simulink model "EMB_CVT"  (R2023a)
settings: Solver=VariableStepAuto  StartTime=0.0  StopTime=200.0  RelTol=1e-3
undefined symbols (not defined in the file): controller, sigbuilder_block
libraries: fl_lib x19, sdl_lib x9, nesl_utility x8, simulink x1, slpidlib x1, autolibshared x1, batteryecm_lib x1, BatteryEstimators x1, ee_lib x1
settings Model: Creator=Rohan  LastModifiedBy=Rohan

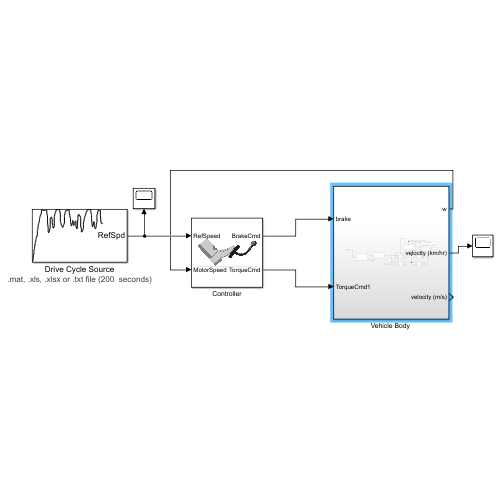
[thumbnail: Simulink's stored preview of the top-level diagram]
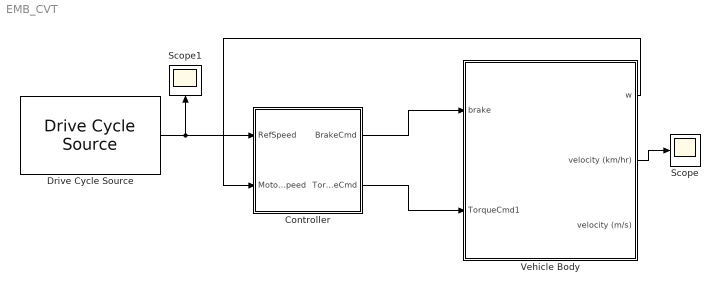
== system EMB_CVT ==
  Controller : Subsystem  VariantControl=a==1
      mask Display: image('$imagefile'); % Use "Edit Image" on toolstrip to change.
  Drive Cycle Source : autolibshared/Drive Cycle Source  cycleVar=.mat, .xls, .xlsx or .txt file  fileVar=D:\BAJA Battery\Day2 (1)\Day2\1_drive_cycle\driveCycleb.mat  tfinal="200  seconds"  cycleRepeat=off  outAccPort=off  outGearPort=off  gearList=No gear data  t_wot1=5  xdot_woto=0  xdot_wot1=30  t_wot2=20  xdot_wot2=0  t_wotend=30  srcUnit=m/s  outUnit=m/s  srcAccUnit=m/s/s  outAccUnit=m/s^2  dt=0  aMode=1  faultOption=off  velBnd=2  velBndUnit=mph  inUnit=m/s  timeBnd=1  failOption=off  stopSim=off  maxFaultCnt=10  maxFaultTime=2  maxTotFaultTime=15  traceOption=off  dtTrace=1  traceWindow=10  lastDCname=Custom Data Set  lastOutUnit=mph  lastDT=0  lastTB=1  lastSB=2  forceCalcBound=off
  Scope : Scope
  Scope1 : Scope
  "Vehicle Body " : Subsystem
  wires:
  Controller/2(TorqueCmd) -> "Vehicle Body "/2(TorqueCmd1)
  "Vehicle Body "/2(velocity (km/hr)) -> Scope/1
  Controller/1(BrakeCmd) -> "Vehicle Body "/1(brake)
  Drive Cycle Source/1 -> Controller/1(RefSpeed), Scope1/1
  "Vehicle Body "/1(w) -> Controller/2(MotorSpeed)

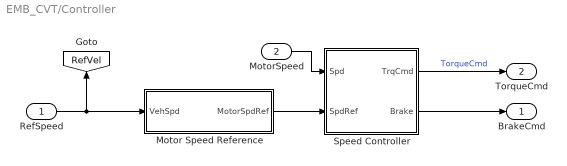
== system EMB_CVT/Controller ==
  RefSpeed : Inport
  MotorSpeed : Inport  Port=2
  Motor Speed Reference : Subsystem
  Speed Controller : Subsystem
      settings: PortSchema="{\"entries\":[{\"content\":{\"sides\":[{\"content\":{\"connectorIds\":[\"Out1\",\"Out2\"]},\"type\":\"ConnectorPlacement.EquallySpacedRectSide\",\"uuid\":\"12b9f2c9-2b28-451b-ad36-7fe4150db485\"},{\"content\":{\"connectorIds\":[\"In1\",\"In2\"],\"side\":\"RIGHT\"},\"type\":\"ConnectorPlacement.EquallySpacedRectSide\",\"uuid\":\"c0fdf9a4-483a-4ddc-b663-6299fcc79327\"},{\"content\":{\"connectorIds\":[],\"side\":\"TOP\"},\"type\":\"ConnectorPlacement.EquallySpacedRectSide\",\"uuid\":\"3f20082e-8487-45e3-9fd7-d6d75741df4d\"}]},\"type\":\"ConnectorPlacement.EquallySpacedConnector\",\"uuid\":\"9361cdd3-74d8-46ee-ae7f-e2dde5d31ed1\"}],\"packageUris\":[\"http://schema.mathworks.com/mf0/Connector/R2020b\"],\"version\":\"1.0\"}"
  BrakeCmd : Outport
  TorqueCmd : Outport  Port=2
  tag scope: RefVel=global
  wires:
  Speed Controller/2(Brake) -> BrakeCmd/1
  Motor Speed Reference/1(MotorSpdRef) -> Speed Controller/2(SpdRef)
  MotorSpeed/1 -> Speed Controller/1(Spd)
  Speed Controller/1(TrqCmd) -> TorqueCmd/1  "TorqueCmd"
  RefSpeed/1 -> Motor Speed Reference/1(VehSpd), [RefVel]

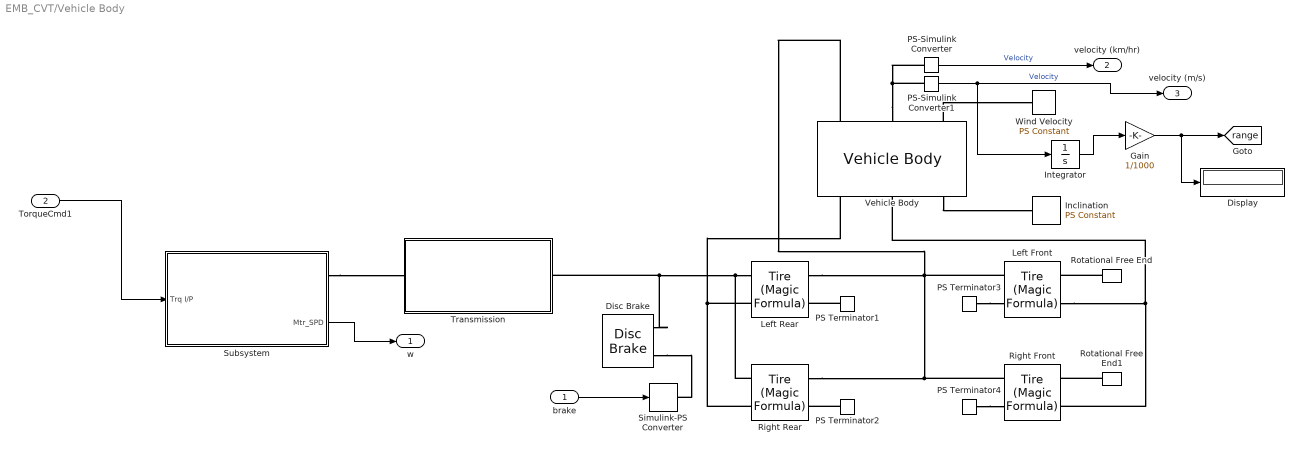
== system EMB_CVT/Vehicle Body  ==
  brake : Inport
  TorqueCmd1 : Inport  Port=2
  Disc Brake : sdl_lib/Brakes & Detents/Rotational/Disc Brake  r_mean=brake.padRadius mm  bore=brake.cylinderBore mm  n_pads=2  thermal_port=simscape.enum.thermaleffects.omit  mu_static=brake.sf  mu_coulomb=brake.cf  temperature_TLU=[280, 300, 320] K  mu_static_TLU=[.9, .8, .7]  mu_coulomb_TLU=[.8, .7, .6]  brkwy_vel=brake.frictionVel rad/s  visc_coef=0 N*m*s/rad  enable_faults=simscape.enum.onoff.off  faulted_pressure=0 bar  external_fault=simscape.enum.onoff.off  temporal_fault=simscape.enum.onoff.off  fault_time=5 s  report_fault=simscape.enum.assert.action.none  thermal_mass=50 kJ/K  temperature_specify=off  temperature_priority=High  temperature=300 K  temperature_nominal_specify=off  temperature_nominal_unit=K  temperature_nominal_value=1
  Display : Display
  Gain : Gain  Gain=1/1000
  Inclination : fl_lib/Physical Signals/Sources/PS Constant  constant=0
  Integrator : Integrator
  Left Front : sdl_lib/Tires & Vehicles/Tire (Magic Formula)  parameterization=sdl.enum.magic_tire_model.constant  F_z1=3000 N  F_x1=3500 N  kappa1=10  B_m=vehicle.tireBCoeff  C_m=vehicle.tireCCoeff  D_m=vehicle.tireDCoeff  E_m=vehicle.tireECoeff  fz0=4000 N  p_Cx=1.685  p_Dx=[1.21, -.037]  p_Ex=[.344, .095, -.02, 0]  p_Kx=[21.51, -.163, .245]  p_Hx=[-.002, .002]  p_Vx=[0, 0]  rolling_radius_model=sdl.enum.RollingRadiusParameterization.Constant  r_e=vehicle.tireRollingRadius m  r_0=0.3 m  breff=8.39  dreff=0.26  freff=0.074  q_re0=0.99  q_v1=0.008  longvl=17 m/s  cz=5e5 N/m  model_resistance=1  resistance_model=1  coeff=0.005  p_tire=250e3 Pa  alpha=-0.003  beta=0.97  coeff_a=84e-4  coeff_b=6.2e-4 s/m  coeff_c=1.6e-4 s^2/m^2  p_tire0=240e3 Pa  fz0_resistance=4000 N  vH0=16 m/s  q_Sy=[.0082, 0, .0014, .001, 0, 0, 1.08, -.5]  v_thr=0.001 m/s  enable_scaling_coefficients=false  lfzO=1  lcx=1  lmux=1  lex=1  lkx=1  lhx=1  lvx=1  lmy=1  model_compliance=0  stiffness=1e6 N/m  damping=1000 N/(m/s)  model_inertia=1  inertia=1e-2 kg*m^2  initial_velocity=0 rpm  vxlow=0.1 m/s  v_tr_thr=0.1*(0.1) m/s  kpumin=-1e5  kpumax=1e5
  Left Rear : sdl_lib/Tires & Vehicles/Tire (Magic Formula)  parameterization=sdl.enum.magic_tire_model.constant  F_z1=3000 N  F_x1=3500 N  kappa1=10  B_m=vehicle.tireBCoeff  C_m=vehicle.tireCCoeff  D_m=vehicle.tireDCoeff  E_m=vehicle.tireECoeff  fz0=4000 N  p_Cx=1.685  p_Dx=[1.21, -.037]  p_Ex=[.344, .095, -.02, 0]  p_Kx=[21.51, -.163, .245]  p_Hx=[-.002, .002]  p_Vx=[0, 0]  rolling_radius_model=sdl.enum.RollingRadiusParameterization.Constant  r_e=vehicle.tireRollingRadius m  r_0=0.3 m  breff=8.39  dreff=0.26  freff=0.074  q_re0=0.99  q_v1=0.008  longvl=17 m/s  cz=5e5 N/m  model_resistance=1  resistance_model=1  coeff=0.005  p_tire=250e3 Pa  alpha=-0.003  beta=0.97  coeff_a=84e-4  coeff_b=6.2e-4 s/m  coeff_c=1.6e-4 s^2/m^2  p_tire0=240e3 Pa  fz0_resistance=4000 N  vH0=16 m/s  q_Sy=[.0082, 0, .0014, .001, 0, 0, 1.08, -.5]  v_thr=0.001 m/s  enable_scaling_coefficients=false  lfzO=1  lcx=1  lmux=1  lex=1  lkx=1  lhx=1  lvx=1  lmy=1  model_compliance=0  stiffness=1e6 N/m  damping=1000 N/(m/s)  model_inertia=1  inertia=1e-2 kg*m^2  initial_velocity=0 rpm  vxlow=0.1 m/s  v_tr_thr=0.1*(0.1) m/s  kpumin=-1e5  kpumax=1e5
  PS Terminator{1..4} (4 alike) : fl_lib/Physical Signals/Sinks/PS Terminator
  PS-Simulink Converter : nesl_utility/PS-Simulink Converter  PhysicalDomain=network_engine_domain  SubClassName=ps_output  LeftPortType=input  RightPortType=output  PseudoPeriodic=off  Frequencies=[]  VectorFormat=1-D array  Unit=km/hr  AffineConversion=off
  PS-Simulink Converter1 : nesl_utility/PS-Simulink Converter  PhysicalDomain=network_engine_domain  SubClassName=ps_output  LeftPortType=input  RightPortType=output  PseudoPeriodic=off  Frequencies=[]  VectorFormat=1-D array  Unit=m/s  AffineConversion=off
  Right Front : sdl_lib/Tires & Vehicles/Tire (Magic Formula)  parameterization=sdl.enum.magic_tire_model.constant  F_z1=3000 N  F_x1=3500 N  kappa1=10  B_m=vehicle.tireBCoeff  C_m=vehicle.tireCCoeff  D_m=vehicle.tireDCoeff  E_m=vehicle.tireECoeff  fz0=4000 N  p_Cx=1.685  p_Dx=[1.21, -.037]  p_Ex=[.344, .095, -.02, 0]  p_Kx=[21.51, -.163, .245]  p_Hx=[-.002, .002]  p_Vx=[0, 0]  rolling_radius_model=sdl.enum.RollingRadiusParameterization.Constant  r_e=vehicle.tireRollingRadius m  r_0=0.3 m  breff=8.39  dreff=0.26  freff=0.074  q_re0=0.99  q_v1=0.008  longvl=17 m/s  cz=5e5 N/m  model_resistance=1  resistance_model=1  coeff=0.005  p_tire=250e3 Pa  alpha=-0.003  beta=0.97  coeff_a=84e-4  coeff_b=6.2e-4 s/m  coeff_c=1.6e-4 s^2/m^2  p_tire0=240e3 Pa  fz0_resistance=4000 N  vH0=16 m/s  q_Sy=[.0082, 0, .0014, .001, 0, 0, 1.08, -.5]  v_thr=0.001 m/s  enable_scaling_coefficients=false  lfzO=1  lcx=1  lmux=1  lex=1  lkx=1  lhx=1  lvx=1  lmy=1  model_compliance=0  stiffness=1e6 N/m  damping=1000 N/(m/s)  model_inertia=1  inertia=1e-2 kg*m^2  initial_velocity=0 rpm  vxlow=0.1 m/s  v_tr_thr=0.1*(0.1) m/s  kpumin=-1e5  kpumax=1e5
  Right Rear : sdl_lib/Tires & Vehicles/Tire (Magic Formula)  parameterization=sdl.enum.magic_tire_model.constant  F_z1=3000 N  F_x1=3500 N  kappa1=10  B_m=vehicle.tireBCoeff  C_m=vehicle.tireCCoeff  D_m=vehicle.tireDCoeff  E_m=vehicle.tireECoeff  fz0=4000 N  p_Cx=1.685  p_Dx=[1.21, -.037]  p_Ex=[.344, .095, -.02, 0]  p_Kx=[21.51, -.163, .245]  p_Hx=[-.002, .002]  p_Vx=[0, 0]  rolling_radius_model=sdl.enum.RollingRadiusParameterization.Constant  r_e=vehicle.tireRollingRadius m  r_0=0.3 m  breff=8.39  dreff=0.26  freff=0.074  q_re0=0.99  q_v1=0.008  longvl=17 m/s  cz=5e5 N/m  model_resistance=1  resistance_model=1  coeff=0.005  p_tire=250e3 Pa  alpha=-0.003  beta=0.97  coeff_a=84e-4  coeff_b=6.2e-4 s/m  coeff_c=1.6e-4 s^2/m^2  p_tire0=240e3 Pa  fz0_resistance=4000 N  vH0=16 m/s  q_Sy=[.0082, 0, .0014, .001, 0, 0, 1.08, -.5]  v_thr=0.001 m/s  enable_scaling_coefficients=false  lfzO=1  lcx=1  lmux=1  lex=1  lkx=1  lhx=1  lvx=1  lmy=1  model_compliance=0  stiffness=1e6 N/m  damping=1000 N/(m/s)  model_inertia=1  inertia=1e-2 kg*m^2  initial_velocity=0 rpm  vxlow=0.1 m/s  v_tr_thr=0.1*(0.1) m/s  kpumin=-1e5  kpumax=1e5
  Rotational Free End : fl_lib/Mechanical/Rotational Elements/Rotational Free End  w_specify=off  w_priority=None  w=0 rad/s  w_nominal_specify=off  w_nominal_unit=rad/s  w_nominal_value=1
  Rotational Free End1 : fl_lib/Mechanical/Rotational Elements/Rotational Free End  w_specify=off  w_priority=None  w=0 rad/s  w_nominal_specify=off  w_nominal_unit=rad/s  w_nominal_value=1
  Simulink-PS Converter : nesl_utility/Simulink-PS Converter  PhysicalDomain=network_engine_domain  SubClassName=ps_input  LeftPortType=input  RightPortType=output  PseudoPeriodic=off  Frequencies=[]  NoiseDistribution=none  NoiseParameters=[]  Unit=N/m^2  AffineConversion=off  FilteringAndDerivatives=filter  SimscapeFilterOrder=2  InputFilterTimeConstant=0.001  UdotUserProvided=1
  Subsystem : Subsystem
      settings: PortSchema="{\"entries\":[{\"content\":{\"sides\":[{\"content\":{\"connectorIds\":[\"In1\"]},\"type\":\"ConnectorPlacement.EquallySpacedRectSide\",\"uuid\":\"a8b1f416-e8b0-4c0a-8f46-8c70d4c0ad6f\"},{\"content\":{\"connectorIds\":[\"RConn1\",\"Out1\"],\"side\":\"RIGHT\"},\"type\":\"ConnectorPlacement.EquallySpacedRectSide\",\"uuid\":\"f31562b3-4fb8-47fa-b272-1277153c0f5f\"},{\"content\":{\"side\":\"TOP\"},\"type\":\"ConnectorPlacement.EquallySpacedRectSide\",\"uuid\":\"367d0b97-d35b-412e-9cb2-5cff6624febc\"}]},\"type\":\"ConnectorPlacement.EquallySpacedConnector\",\"uuid\":\"bebd6450-d495-493e-a389-2977d92ebb5e\"}],\"packageUris\":[\"http://schema.mathworks.com/mf0/Connector/R2020b\"],\"version\":\"1.0\"}"
  Transmission : Subsystem
  Vehicle Body : sdl_lib/Tires & Vehicles/Vehicle Body  mass=vehicle.mass kg  n_w=vehicle.numAxle  x_f=vehicle.cgFrontAxle m  x_r=vehicle.cgRearAxle m  y_c=vehicle.cgGround m  mass_var=simscape.enum.onoff.off  g=9.81 m/s^2  liftoff_warning=0  area=.735482 m^2  Cd=1.92  rho=1.18 kg/m^3  model_pitch=0  inertia=4000 kg*m^2  suspension_model=1  k_f=1e4 N/m  b_f=1e4 N/(m/s)  k_r=1e4 N/m  b_r=1e4 N/(m/s)  k_f_TLU=[-2000, -1000, 0, 1000, 2000] N  x_f_TLU=[-.4, -.2, 0, .2, .4] m  b_f_TLU=[-200, -100, 0, 100, 200] N  v_f_TLU=[-4, -2, 0, 2, 4] m/s  k_r_TLU=[-2000, -1000, 0, 1000, 2000] N  x_r_TLU=[-.4, -.2, 0, .2, .4] m  b_r_TLU=[-200, -100, 0, 100, 200] N  v_r_TLU=[-4, -2, 0, 2, 4] m/s  interp_method=simscape.enum.interpolation.linear  extrap_method=simscape.enum.extrapolation.linear  model_hardstop=0  upper_bound_f=.25 m  lower_bound_f=-.25 m  stop_k_f=1e6 N/m  stop_b_f=150 N/(m/s)  upper_bound_r=.25 m  lower_bound_r=-.25 m  stop_k_r=1e6 N/m  stop_b_r=150 N/(m/s)  initial_pitch=0 rad  initial_pitch_rate=0 rad/s  v_specify=on  v_priority=High  v=0 m/s  v_nominal_specify=off  v_nominal_unit=m/s  v_nominal_value=1
  Wind Velocity : fl_lib/Physical Signals/Sources/PS Constant  constant=0
  w : Outport
  velocity (km/hr) : Outport  Port=2
  velocity (m/s) : Outport  Port=3
  tag scope: range=global
  wires:
  Integrator/1 -> Gain/1
  PS-Simulink Converter1/1 -> Integrator/1, velocity (m/s)/1  "Velocity"
  brake/1 -> Simulink-PS Converter/1
  PS-Simulink Converter/1 -> velocity (km/hr)/1  "Velocity"
  Gain/1 -> Display/1, [range]
  TorqueCmd1/1 -> Subsystem/1(Trq I/P)
  Subsystem/1(Mtr_SPD) -> w/1
  connections:
  Vehicle Body/RConn2 -- Right Front/LConn1 -- Left Front/LConn1
  Vehicle Body/LConn2 -- PS-Simulink Converter/LConn1 -- PS-Simulink Converter1/LConn1
  Right Front/RConn2 -- Vehicle Body/LConn1 -- Left Rear/RConn2 -- Left Front/RConn2 -- Right Rear/RConn2
  Vehicle Body/RConn1 -- Left Rear/LConn1 -- Right Rear/LConn1
  PS Terminator1/LConn1 -- Left Rear/RConn1
  Vehicle Body/LConn3 -- Wind Velocity/RConn1
  Vehicle Body/RConn3 -- Inclination/RConn1
  Disc Brake/LConn1 -- Simulink-PS Converter/RConn1
  PS Terminator3/LConn1 -- Left Front/RConn1
  PS Terminator2/LConn1 -- Right Rear/RConn1
  Rotational Free End/LConn1 -- Left Front/LConn2
  PS Terminator4/LConn1 -- Right Front/RConn1
  Rotational Free End1/LConn1 -- Right Front/LConn2
  Right Rear/LConn2 -- Disc Brake/LConn2 -- Transmission/RConn1 -- Left Rear/LConn2
  Subsystem/RConn1 -- Transmission/LConn1

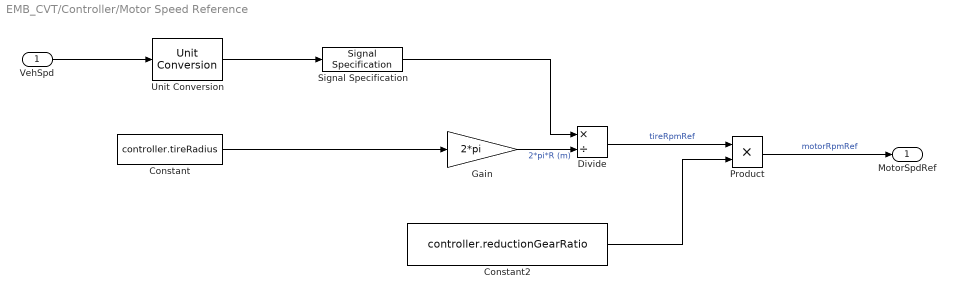
== system EMB_CVT/Controller/Motor Speed Reference ==
  VehSpd : Inport  Unit=km/hr
  Constant : Constant  Value=controller.tireRadius
  Constant2 : Constant  Value=controller.reductionGearRatio
  Divide : Product  Inputs=*/
  Gain : Gain  Gain=2*pi
  Product : Product
  Signal Specification : SignalSpecification  Unit=m/min
  Unit Conversion : UnitConversion
  MotorSpdRef : Outport  Unit=rpm  VectorParamsAs1DForOutWhenUnconnected=off
  wires:
  Product/1 -> MotorSpdRef/1  "motorRpmRef"
  Constant2/1 -> Product/2
  Divide/1 -> Product/1  "tireRpmRef"
  Gain/1 -> Divide/2  "2*pi*R (m)"
  Signal Specification/1 -> Divide/1
  Unit Conversion/1 -> Signal Specification/1
  VehSpd/1 -> Unit Conversion/1
  Constant/1 -> Gain/1

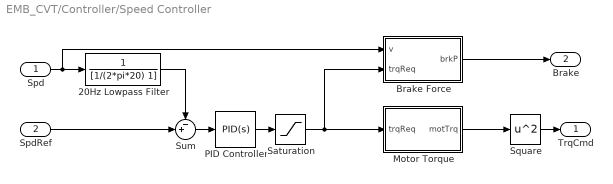
== system EMB_CVT/Controller/Speed Controller ==
  Spd : Inport  Unit=rpm
  SpdRef : Inport  Port=2  Unit=rpm
  20Hz Lowpass Filter : TransferFcn  Denominator=[1/(2*pi*20) 1]
  Brake Force : Subsystem
  Motor Torque : Subsystem
  PID Controller : slpidlib/PID Controller  Controller=PID  Form=Parallel  TimeDomain=Continuous-time  UseExternalTs=off  SampleTime=-1  IntegratorMethod=Forward Euler  FilterMethod=Forward Euler  ControllerParametersSource=internal  P=1  I=1  UseKiTs=off  D=0  N=100  UseFilter=on  TunerSelectOption=Transfer Function Based (PID Tuner App)  InitialConditionSource=internal  InitialConditionForIntegrator=0  InitialConditionForFilter=0  DifferentiatorICPrevScaledInput=0  ExternalReset=none  TrackingMode=off  Kt=1  LimitOutput=off  SatLimitsSource=internal  UpperSaturationLimit=inf  LowerSaturationLimit=-inf  LinearizeAsGain=on  AntiWindupMode=none  Kb=1  LimitIntegrator=off  UpperIntegratorSaturationLimit=inf  LowerIntegratorSaturationLimit=-inf  POutMin=[]  POutMax=[]  IOutMin=[]  IOutMax=[]  DOutMin=[]  DOutMax=[]  NOutMin=[]  NOutMax=[]  SumOutMin=[]  SumOutMax=[]  SaturationOutMin=[]  SaturationOutMax=[]  PParamMin=[]  PParamMax=[]  IParamMin=[]  IParamMax=[]  DParamMin=[]  DParamMax=[]  NParamMin=[]  NParamMax=[]  KbParamMin=[]  KbParamMax=[]  KtParamMin=[]  KtParamMax=[]  KbOutMin=[]  KbOutMax=[]  KtOutMin=[]  KtOutMax=[]  IntegratorOutMin=[]  IntegratorOutMax=[]  FilterOutMin=[]  FilterOutMax=[]  SumI1OutMin=[]  SumI1OutMax=[]  SumI2OutMin=[]  SumI2OutMax=[]  SumI3OutMin=[]  SumI3OutMax=[]  SumI4OutMin=[]  SumI4OutMax=[]  SumDOutMin=[]  SumDOutMax=[]  DifferentiatorOutMin=[]  DifferentiatorOutMax=[]  FilterDiffOutCoefMin=[]  FilterDiffOutCoefMax=[]  ReciprocalOutMin=[]  ReciprocalOutMax=[]  SumDenOutMin=[]  SumDenOutMax=[]  SumNumOutMin=[]  SumNumOutMax=[]  DivideOutMin=[]  DivideOutMax=[]  UdiffTsProdOutMin=[]  UdiffTsProdOutMax=[]  NTsProdOutMin=[]  NTsProdOutMax=[]  UintegralTsProdOutMin=[]  UintegralTsProdOutMax=[]  UngainTsProdOutMin=[]  UngainTsProdOutMax=[]  ClampingZeroOutDataTypeStr=Inherit: Inherit via back propagation  ClampingZeroOutMin=[]  ClampingZeroOutMax=[]  FilterDenConstantOutDataTypeStr=Inherit: Inherit via back propagation  FilterDenConstantOutMin=[]  FilterDenConstantOutMax=[]  PCopyOutDataTypeStr=Inherit: Inherit via back propagation  PCopyOutMin=[]  PCopyOutMax=[]  NCopyOutDataTypeStr=Inherit: Inherit via back propagation  NCopyOutMin=[]  NCopyOutMax=[]  IntegratorContinuousStateAttributes=''  IntegratorStateMustResolveToSignalObject=off  IntegratorRTWStateStorageClass=Auto  FilterContinuousStateAttributes=''  FilterStateMustResolveToSignalObject=off  FilterRTWStateStorageClass=Auto  ParallelPVariant=InternalParameters  IdealPVariant=Disabled  IVariant=InternalParameters  DVariant=InternalParameters  IntegratorVariant=Continuous  SatVariant=Disabled  AWVariant=Passthrough  PCopyVariant=Disabled  TRVariant=Disabled  FdbkBlocksVariant=Forward  IdealPFdbkVariant=Disabled  SatFdbkVariant=Disabled  DerivativeFilterVariant=ContFilter  NVariant=InternalParameters  NCopyVariant=Disabled  FilterICVariant=InternalICsFilter  IntegratorICVariant=InternalICs  ExternalResetVariant=Disabled  TRSumVariant=Passthrough  SumFdbkVariant=Disabled  SumVariant=Sum_PID  TsampFilterVariant=InternalTs  TsampNgainVariant=Passthrough  TsampIntegralVariant=Disabled_SignalSpec  ExternalSaturationOutDataTypeStr=Inherit: Same as second input
  Saturation : Saturate  UpperLimit=35  LowerLimit=-35
      settings: AttributesFormatString=|
      | %<UpperLimit>
      | %<LowerLimit>
  Square : Math  Operator=square
  Sum : Sum  Inputs=-+|
  TrqCmd : Outport  Unit=N*m  VectorParamsAs1DForOutWhenUnconnected=off
      settings: AttributesFormatString=%<Unit>
  Brake : Outport  Port=2  VectorParamsAs1DForOutWhenUnconnected=off
      settings: AttributesFormatString=%<Unit>
  wires:
  Saturation/1 -> Motor Torque/1(trqReq), Brake Force/2(trqReq)
  SpdRef/1 -> Sum/2
  PID Controller/1 -> Saturation/1
  Sum/1 -> PID Controller/1
  Spd/1 -> Brake Force/1(v), 20Hz Lowpass Filter/1
  Brake Force/1(brkP) -> Brake/1
  20Hz Lowpass Filter/1 -> Sum/1
  Square/1 -> TrqCmd/1
  Motor Torque/1(motTrq) -> Square/1

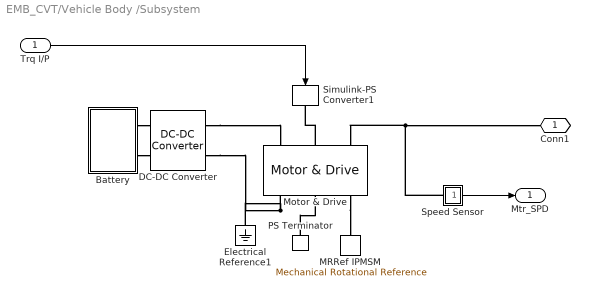
== system EMB_CVT/Vehicle Body /Subsystem ==
  Trq I/P : Inport
  Battery : Subsystem
  DC-DC Converter : ee_lib/Semiconductors & Converters/Converters/DC-DC Converter  Vref_option=ee.enum.converters.voltageref.internal  v_ref=converter.outputVoltage V  P_rated=converter.outputPower kW  droop_enabled=true  droop_param=ee.enum.converters.droop.percent  droop=0.1 V/A  droop_percent=converter.droopPercent  Vref_droop=10 V  reversible=ee.enum.converters.directionality.bidirectional  G_diode=1e-8 1/Ohm  P_fixed=1 W  losses_option=ee.enum.converters.lossesOption.proportionalToSquaredCurrent  eff_rated=80  tableOption=ee.enum.converters.lossTableOptionThermal.currentTemp  i_eff_vec=[-2, -1, 1, 2] A  v_eff_vec=[15, 30, 45] V  eff_vec=[66, 76, 80, 74]  eff_2D_table=[66, 66, 66; 76, 76, 76; 80, 80, 80; 74, 74, 74]  model_dynamics=ee.enum.converters.dynamics.no  tau=0.02 s  v_ini=10 V  v1_min=1 V  R1=1000 Ohm  R2=1000 Ohm  enable_fault=simscape.enum.onoff.off  fault_condition=ee.enum.faults.faultInputCondition.greaterThan  fault_threshold=0.5  T_eff_vec=[280, 300, 320] K  eff_3D_table=repmat([66; 76; 80; 74], 1, 3, 3)  thermal_mass=100 J/K  initial_temperature=298.15 K
      settings: InternalSimscapePortConfiguration="{\"Bottom\":[],\"Left\":[{\"id\":\"p1\",\"label\":\"1+\",\"type\":\"foundation.electrical.electrical\"},{\"id\":\"n1\",\"label\":\"1-\",\"type\":\"foundation.electrical.electrical\"}],\"Right\":[{\"id\":\"p2\",\"label\":\"2+\",\"type\":\"foundation.electrical.electrical\"},{\"id\":\"n2\",\"label\":\"2-\",\"type\":\"foundation.electrical.electrical\"}],\"Top\":[]}"
  Electrical Reference1 : fl_lib/Electrical/Electrical Elements/Electrical Reference
  MRRef IPMSM : fl_lib/Mechanical/Rotational Elements/Mechanical Rotational Reference
  Motor & Drive : sdl_lib/Engines & Motors/Motor & Drive  torque_max=motor.maxTorque N*m  power_max=motor.maxPower kW  Tc=motor.torqueTc s  eff=motor.overallEfficiency  w_eff=motor.speedatEff rpm  T_eff=motor.torqueatEff N*m  thermal_port=simscape.enum.thermaleffects.omit  thermal_mass=10 J/K  temperature_specify=on  temperature_priority=High  temperature=5 degC  temperature_nominal_specify=off  temperature_nominal_unit=K  temperature_nominal_value=1
      settings: InternalSimscapePortConfiguration="{\"Bottom\":[],\"Left\":[{\"id\":\"Vp\",\"label\":\"+\",\"type\":\"foundation.electrical.electrical\"},{\"id\":\"Tr\",\"label\":\"Tr\",\"type\":\"input\"},{\"id\":\"R\",\"label\":\"R\",\"type\":\"foundation.mechanical.rotational.rotational\"}],\"Right\":[{\"id\":\"Vm\",\"label\":\"-\",\"type\":\"foundation.electrical.electrical\"},{\"id\":\"Omega\",\"label\":\"w\",\"type\":\"output\"},{\"id\":\"C\",\"label\":\"C\",\"type\":\"foundation.mechanical.rotational.rotational\"}],\"Top\":[]}"
  PS Terminator : fl_lib/Physical Signals/Sinks/PS Terminator
  Simulink-PS Converter1 : nesl_utility/Simulink-PS Converter  PhysicalDomain=network_engine_domain  SubClassName=ps_input  LeftPortType=input  RightPortType=output  PseudoPeriodic=off  Frequencies=[]  NoiseDistribution=none  NoiseParameters=[]  Unit=N*m  AffineConversion=off  FilteringAndDerivatives=zero  SimscapeFilterOrder=1  InputFilterTimeConstant=.001  UdotUserProvided=0
  Speed Sensor : Subsystem
      mask Display: disp('w')
  Conn1 : PMIOPort  Side=Right
  Mtr_SPD : Outport
  wires:
  Speed Sensor/1(w) -> Mtr_SPD/1
  Trq I/P/1 -> Simulink-PS Converter1/1
  connections:
  Speed Sensor/LConn1 -- Conn1/RConn1 -- Motor & Drive/LConn3
  PS Terminator/LConn1 -- Motor & Drive/RConn2
  Motor & Drive/RConn3 -- MRRef IPMSM/LConn1
  Motor & Drive/LConn2 -- Simulink-PS Converter1/RConn1
  Battery/RConn2 -- DC-DC Converter/LConn2
  Battery/RConn1 -- DC-DC Converter/LConn1
  DC-DC Converter/RConn1 -- Motor & Drive/LConn1
  Motor & Drive/RConn1 -- DC-DC Converter/RConn2 -- Electrical Reference1/LConn1

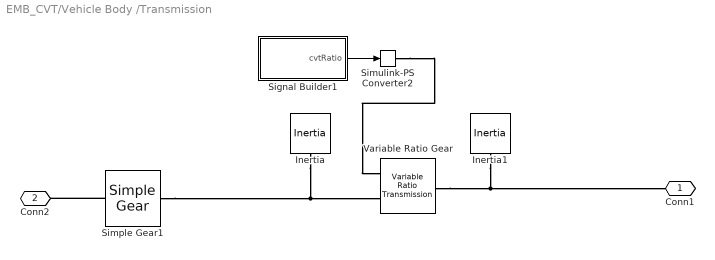
== system EMB_CVT/Vehicle Body /Transmission ==
  Inertia : fl_lib/Mechanical/Rotational Elements/Inertia  inertia=0.1 kg*m^2  num_ports=foundation.enum.numPorts2.one  w_specify=off  w_priority=High  w=0 rad/s  w_nominal_specify=off  w_nominal_unit=rad/s  w_nominal_value=1  t_specify=off  t_priority=None  t=0 N*m  t_nominal_specify=off  t_nominal_unit=N*m  t_nominal_value=1
  Inertia1 : fl_lib/Mechanical/Rotational Elements/Inertia  inertia=0.1 kg*m^2  num_ports=foundation.enum.numPorts2.one  w_specify=off  w_priority=High  w=0 rad/s  w_nominal_specify=off  w_nominal_unit=rad/s  w_nominal_value=1  t_specify=off  t_priority=None  t=0 N*m  t_nominal_specify=off  t_nominal_unit=N*m  t_nominal_value=1
  Signal Builder1 : Subsystem  Tag=STV Subsys  LoadFcn=sigbuilder_block('load');  StartFcn=sigbuilder_block('start');  StopFcn=sigbuilder_block('stop');  ClipboardFcn=sigbuilder_block('clipboard');  mask(Sigbuilder block){tuvar=[0:10]}
      mask help: Simulink:masks:SigbuilderBlock_MD
      mask init:
      | if ~strcmp(get_param(bdroot(gcbh),'SimulationStatus'),'stopped') tuvar = sigbuilder_block('maskInit'); end
      settings: CopyFcn=sigbuilder_block('copy');  DeleteFcn=sigbuilder_block('delete');  ModelCloseFcn=sigbuilder_block('modelClose');  PreSaveFcn=sigbuilder_block('preSave');  PauseFcn=sigbuilder_block('pause');  ContinueFcn=sigbuilder_block('continue');  NameChangeFcn=sigbuilder_block('namechange');  OpenFcn=sigbuilder_block('open',[5.4 36 1141.2 516.6 ]);  CloseFcn=sigbuilder_block('close');
      mask Display: plot(0, 0, 100, 100,[2, 2, 32, 32, 2], [68, 8, 8, 68, 68],[32, 2], [38, 38], [32, 19, 2],[53, 60, 44], [32, 17, 17, 2],[16, 16, 31, 31]);txt = getActiveGroup(gcbh);text(2, 100, txt,'verticalAlignment', 'top');
  Simple Gear1 : sdl_lib/Gears/Simple Gear  ratio=motor.gear  rotation_direction=sdl.enum.shaftOutputDirection.same  friction_model=sdl.enum.gear_efficiencies_load.off  T_noload=0.1 N*m  T_nom=5 N*m  efficiency_nom=0.8  efficiency=0.8  temperature_TLU=[280, 300, 320] K  load_TLU=[1, 5, 10] N*m  efficiency_TLU=[.95, .9, .85]  efficiency_TLU2=[.85, .8, .75; .95, .9, .85; .85, .8, .7]  w_thr=0.01 rad/s  pwr_thr=0.001 W  enable_backlash=false  hardstop_model=simscape.enum.hardstop.smooth  backlash_distance=1e-3 mm  r_base=0.1 m  transition=1e-4 mm  backlash_stiffness=1e7 N/m  backlash_damping=1e6 N*s/m  coeff_rest=0  v_tol=0.001 m/s  f_tol=0 N  mu_visc=[0, 0] N*m/(rad/s)  enable_faults=simscape.enum.onoff.off  efficiency_fault=0.05  external_fault=simscape.enum.onoff.off  temporal_fault=simscape.enum.onoff.off  fault_time=5 s  fault_angles=pi / 12 rad  report_fault=simscape.enum.assert.action.none  thermal_mass=50 J/K  temperature_specify=off  temperature_priority=High  temperature=300 K  temperature_nominal_specify=off  temperature_nominal_unit=K  temperature_nominal_value=1  x_backlash_specify=off  x_backlash_priority=None  x_backlash=0 mm  x_backlash_nominal_specify=off  x_backlash_nominal_unit=mm  x_backlash_nominal_value=1  f_hardstop_specify=off  f_hardstop_priority=None  f_hardstop=0 N  f_hardstop_nominal_specify=off  f_hardstop_nominal_unit=N  f_hardstop_nominal_value=1  v_backlash_specify=off  v_backlash_priority=None  v_backlash=0 m/s  v_backlash_nominal_specify=off  v_backlash_nominal_unit=m/s  v_backlash_nominal_value=1
  Simulink-PS Converter2 : nesl_utility/Simulink-PS Converter  PhysicalDomain=network_engine_domain  SubClassName=ps_input  LeftPortType=input  RightPortType=output  PseudoPeriodic=off  Frequencies=[]  NoiseDistribution=none  NoiseParameters=[]  Unit=1  AffineConversion=off  FilteringAndDerivatives=provide  SimscapeFilterOrder=1  InputFilterTimeConstant=0.001  UdotUserProvided=0
  Variable Ratio Gear : sdl_lib/Couplings & Drives/Variable Ratio Transmission  rotation_direction=3-2*(1)  kp=1e3 N*m/rad  kv=10 N*m/(rad/s)  initial_torque=10 N*m  losses_model=sdl.enum.lossesOffOn.on  efficiency=0.9  w_thr=0.01 rad/s  mu_visc=[ 0 0 ] N*m/(rad/s)  R_specify=off  R_priority=None  R=1  R_nominal_specify=off  R_nominal_unit=1  R_nominal_value=1
      settings: InternalSimscapePortConfiguration="{\"Bottom\":[],\"Left\":[{\"id\":\"ratio\",\"label\":\"r\",\"type\":\"input\"},{\"id\":\"B\",\"label\":\"B\",\"type\":\"foundation.mechanical.rotational.rotational\"}],\"Right\":[{\"id\":\"F\",\"label\":\"F\",\"type\":\"foundation.mechanical.rotational.rotational\"}],\"Top\":[]}"
  Conn1 : PMIOPort  Side=Right
  Conn2 : PMIOPort  Port=2  Side=Left
  wires:
  Signal Builder1/1(cvtRatio) -> Simulink-PS Converter2/1
  connections:
  Simulink-PS Converter2/RConn1 -- Variable Ratio Gear/LConn1
  Inertia/LConn1 -- Simple Gear1/RConn1 -- Variable Ratio Gear/LConn2
  Variable Ratio Gear/RConn1 -- Conn1/RConn1 -- Inertia1/LConn1
  Simple Gear1/LConn1 -- Conn2/RConn1

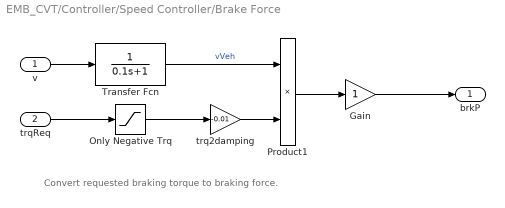
== system EMB_CVT/Controller/Speed Controller/Brake Force ==
  note: Convert requested braking torque to braking force.
  v : Inport
  trqReq : Inport  Port=2
  Gain : Gain
  Only Negative Trq : Saturate  UpperLimit=0  LowerLimit=-inf  ZeroCross=off
  Product1 : Product
  Transfer Fcn : TransferFcn  Denominator=[0.1 1]
  trq2damping : Gain  Gain=-0.01
  brkP : Outport
  wires:
  Gain/1 -> brkP/1
  v/1 -> Transfer Fcn/1
  trqReq/1 -> Only Negative Trq/1
  Transfer Fcn/1 -> Product1/1  "vVeh"
  trq2damping/1 -> Product1/2
  Product1/1 -> Gain/1
  Only Negative Trq/1 -> trq2damping/1

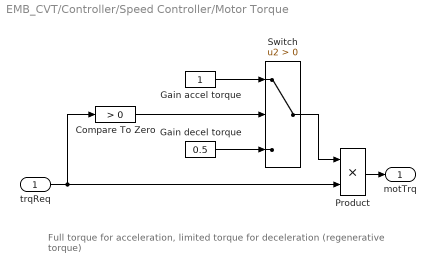
== system EMB_CVT/Controller/Speed Controller/Motor Torque ==
  note: Full torque for acceleration,
      | limited torque for deceleration (regenerative torque)
  trqReq : Inport
  Compare To Zero : simulink/Logic and Bit Operations/Compare To Zero  relop=>  OutDataTypeStr=boolean  ZeroCross=off
  Gain accel torque : Constant
  Gain decel torque : Constant  Value=0.5
  Product : Product
  Switch : Switch  Criteria=u2 > Threshold  SaturateOnIntegerOverflow=off  InputSameDT=off
  motTrq : Outport
  wires:
  Product/1 -> motTrq/1
  trqReq/1 -> Compare To Zero/1, Product/2
  Compare To Zero/1 -> Switch/2
  Gain accel torque/1 -> Switch/1
  Switch/1 -> Product/1
  Gain decel torque/1 -> Switch/3

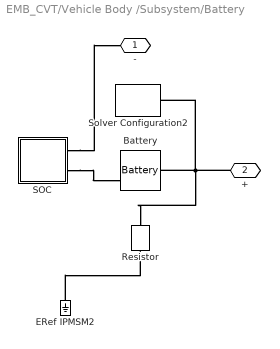
== system EMB_CVT/Vehicle Body /Subsystem/Battery ==
  Battery : batteryecm_lib/Battery  Vnom=battery.nominalVoltage V  prm_dir=simscape.enum.battery.prm_dir.disabled  R1_dis=2 Ohm  R1_ch=2 Ohm  R1=battery.inResistance Ohm  prm_AH=simscape.enum.battery.prm_AH.finite  AH=batter.capacity A*hr  V1=11.5 V  AH1=25 A*hr  prm_R2=simscape.enum.battery.prm_R2.disabled  R2=2000 Ohm  Tmeas=298.15 K  charge_measurement_port=simscape.enum.battery.enable.yes  prm_dyn=simscape.enum.battery.prm_dyn.off  Rp1=0.005 Ohm  tau1=30 s  Rp2=0.005 Ohm  tau2=30 s  Rp3=0.005 Ohm  tau3=30 s  Rp4=0.005 Ohm  tau4=30 s  Rp5=0.005 Ohm  tau5=30 s  prm_fade=simscape.enum.battery.prm_fade.disabled  N_fade=100  AH_fade=45 A*hr  R1_fade=2.02 Ohm  R1_ch_fade=2.02 Ohm  V1_fade=10.35 V  prm_age=simscape.enum.battery.prm_age.disabled  prm_age_OCV=simscape.enum.battery.prm_age_OCV.OCV  OCV_age=0.9  SOC_age=60  Tmeas_age=298.15 K  delta_time_age_vec=[0] d  temperature_age_vec=[273] K  OCV_scaling_age=2.2134e6  OCV_offset_age=1.632e6  temp_exp_age=0.515833569 V  t_exp_age=0.75  Vnom_T2=12 V  R1_T2=2.2 Ohm  R1_T2_dis=2.2 Ohm  R1_T2_ch=2.2 Ohm  V1_T2=11.4 V  R2_T2=2200 Ohm  Rp1_T2=0.005 Ohm  tau1_T2=30 s  Rp2_T2=0.005 Ohm  tau2_T2=30 s  Rp3_T2=0.005 Ohm  tau3_T2=30 s  Rp4_T2=0.005 Ohm  tau4_T2=30 s  Rp5_T2=0.005 Ohm  tau5_T2=30 s  Tmeas2=273.15 K  thermal_port=simscape.enum.thermaleffects.omit  thermal_mass=30000 J/K  i_specify=off  i_priority=None  i=0 A  i_nominal_specify=off  i_nominal_unit=A  i_nominal_value=1  v_specify=off  v_priority=None  v=0 V  v_nominal_specify=off  v_nominal_unit=V  v_nominal_value=1  charge_specify=off  charge_priority=High  charge=50 A*hr  charge_nominal_specify=off  charge_nominal_unit=A*hr  charge_nominal_value=1  num_cycles_specify=off  num_cycles_priority=High  num_cycles=0  num_cycles_nominal_specify=off  num_cycles_nominal_unit=1  num_cycles_nominal_value=1  temperature_specify=off  temperature_priority=High  temperature=298.15 K  temperature_nominal_specify=off  temperature_nominal_unit=K  temperature_nominal_value=1
      settings: InternalSimscapePortConfiguration="{\"Bottom\":[],\"Left\":[{\"id\":\"p\",\"label\":\"+\",\"type\":\"foundation.electrical.electrical\"},{\"id\":\"q\",\"label\":\"q\",\"type\":\"output\"}],\"Right\":[{\"id\":\"n\",\"label\":\"-\",\"type\":\"foundation.electrical.electrical\"}],\"Top\":[]}"
  ERef IPMSM2 : fl_lib/Electrical/Electrical Elements/Electrical Reference
  Resistor : fl_lib/Electrical/Electrical Elements/Resistor  R=1e9 Ohm  i_specify=off  i_priority=None  i=0 A  i_nominal_specify=off  i_nominal_unit=A  i_nominal_value=1  v_specify=off  v_priority=None  v=0 V  v_nominal_specify=off  v_nominal_unit=V  v_nominal_value=1
  SOC : Subsystem
  Solver Configuration2 : nesl_utility/Solver Configuration  PhysicalDomain=network_engine_domain  SubClassName=solver  LeftPortType=input  RightPortType=generic  Tones=[]  Harmonics=[]  SimulateNoise=off  Profile=off  UseLocalSampling=off  EnableSwitchedLinearOptims=on  FrequencyDomain=off  UseCCode=off  RelTol=0.001  AbsTol=1e-06  MinStep=1e-09  ToWorkspace=off  RevertToSquareIcSolve=off  NumHomotopyIterations=100  PhasorMode=off  PhasorModeNumHarmonics=1  ConsistencySolver=NEWTON_FTOL  IndexReductionMethod=DerivativeReplacement  DoDC=off  ResidualTolerance=1e-9  ConsistencyTolSource=GLOBAL  ConsistencyAbsTol=0.001  ConsistencyRelTol=0.001  ConsistencyTolFactor=0.001  UseLocalSolver=on  LocalSolverChoice=NE_BACKWARD_EULER_ADVANCER  ResolveIndetEquations=on  FunctionEvalNumThread=1  LocalSolverSampleTime=1e-03  DoFixedCost=on  MaxNonlinIter=1  MaxModeIter=2  ComputeImpulses=off  ImpulseIterations=2  LinearAlgebra=auto  LinearAlgebraNumThread=0  EquationFormulation=NE_TIME_EF  DelaysMemoryBudget=1024  AutomaticFiltering=on  FilteringTimeConstant=0.001  PartitionStorageMethod=AS_NEEDED  PartitionMemoryBudget=1024  PartitionMethod=FAST
  - : PMIOPort  Side=Right
  + : PMIOPort  Port=2  Side=Right
  connections:
  SOC/RConn1 -- -/RConn1
  +/RConn1 -- Resistor/LConn1 -- Battery/RConn1 -- Solver Configuration2/RConn1
  ERef IPMSM2/LConn1 -- Resistor/RConn1
  SOC/RConn2 -- Battery/LConn1

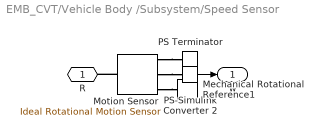
== system EMB_CVT/Vehicle Body /Subsystem/Speed Sensor ==
  Mechanical Rotational Reference1 : fl_lib/Mechanical/Rotational Elements/Mechanical Rotational Reference
  Motion Sensor : fl_lib/Mechanical/Mechanical Sensors/Ideal Rotational Motion Sensor  reference=foundation.enum.MeasurementReference.difference  acceleration_port=false  velocity_port=true  position_port=true  wrap_angle=simscape.enum.onoff.off  offset=0 rad
  PS Terminator : fl_lib/Physical Signals/Sinks/PS Terminator
  PS-Simulink Converter 2 : nesl_utility/PS-Simulink Converter  PhysicalDomain=network_engine_domain  SubClassName=ps_output  LeftPortType=input  RightPortType=output  PseudoPeriodic=off  Frequencies=[]  VectorFormat=1-D array  Unit=rpm  AffineConversion=off
  R : PMIOPort  Side=Left
  w : Outport
  wires:
  PS-Simulink Converter 2/1 -> w/1
  connections:
  Motion Sensor/RConn2 -- PS-Simulink Converter 2/LConn1
  Motion Sensor/RConn1 -- Mechanical Rotational Reference1/LConn1
  Motion Sensor/RConn3 -- PS Terminator/LConn1
  Motion Sensor/LConn1 -- R/RConn1

== system EMB_CVT/Vehicle Body /Transmission/Signal Builder1 ==
  Demux : Demux  Tag=STV Demux  Outputs=1
      settings: DisplayOption=none
  FromWs : FromWorkspace  Tag=STV FromWs  VariableName=tuvar
      SigBuilderData=|
      | common.afterFinalStr = 'Extrapolate'
      | common.sampleTime = 0
      | dataSet.timeRange = [0 20]
      | dataSet.name = 'Group 1'
      | sbobj.Groups.Name = 'Group 1'
      | sbobj.Groups.Signals.Name = 'cvtRatio'
      | sbobj.Groups.Signals.XData = [0 1.69505884503e-08 5.0851765351e-08 8.47529422517e-08 1.58816145203e-07 2.40323907928e-07 2.40323907928e-07 2.60684561726e-07 3.0140586932e-07 3.95584277528e-07 5.48994863555e-07 7.02405449583e-07 ... (1072 elements, 1x1072)]
      | sbobj.Groups.Signals.YData = [3.7 3.7 3.7 3.7 3.7 3.7 3.7 3.7 3.7 3.7 3.7 3.7 ... (1072 elements, 1x1072)]
      | sbobj.Groups.TimeRange = [0 20]
  cvtRatio : Outport  Tag=STV Outport
  wires:
  Demux/1 -> cvtRatio/1
  FromWs/1 -> Demux/1

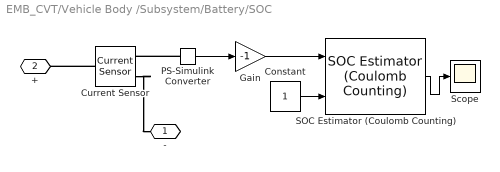
== system EMB_CVT/Vehicle Body /Subsystem/Battery/SOC ==
  Constant : Constant
  Current Sensor : fl_lib/Electrical/Electrical Sensors/Current Sensor
  Gain : Gain  Gain=-1
  PS-Simulink Converter : nesl_utility/PS-Simulink Converter  PhysicalDomain=network_engine_domain  SubClassName=ps_output  LeftPortType=input  RightPortType=output  PseudoPeriodic=off  Frequencies=[]  VectorFormat=1-D array  Unit=A  AffineConversion=off
  SOC Estimator (Coulomb Counting) : BatteryEstimators/SOC Estimator (Coulomb Counting)  AH=batter.capacity  Ts=-1
      settings: LibrarySourceBlock=|
      | batt_sl_lib/Estimators/SOC Estimator
      | (Coulomb Counting)
  Scope : Scope
  - : PMIOPort  Side=Right
  + : PMIOPort  Port=2  Side=Right
  wires:
  PS-Simulink Converter/1 -> Gain/1
  Constant/1 -> SOC Estimator (Coulomb Counting)/2
  Gain/1 -> SOC Estimator (Coulomb Counting)/1
  SOC Estimator (Coulomb Counting)/1 -> Scope/1
  connections:
  PS-Simulink Converter/LConn1 -- Current Sensor/RConn1
  Current Sensor/RConn2 -- -/RConn1
  Current Sensor/LConn1 -- +/RConn1
